simulink model "threeareaIPSnonlinear"  (R2018b)
settings: Solver=VariableStepAuto  StartTime=0.0  StopTime=100  RelTol=1e-3
values from neighbouring files (symbols this model uses):
  optim_param = Best_pos    [main.m]
  w1 = 0.001    [main.m]
  w2 = 0.001    [main.m]
undefined symbols (not defined in the file or in its folder): w3
settings Model: Creator=Orka  LastModifiedBy=Orka
settings SolverCC: ZeroCrossAlgorithm=Adaptive
settings DebuggingCC: MaskedZcDiagnostic=none  IgnoredZcDiagnostic=none

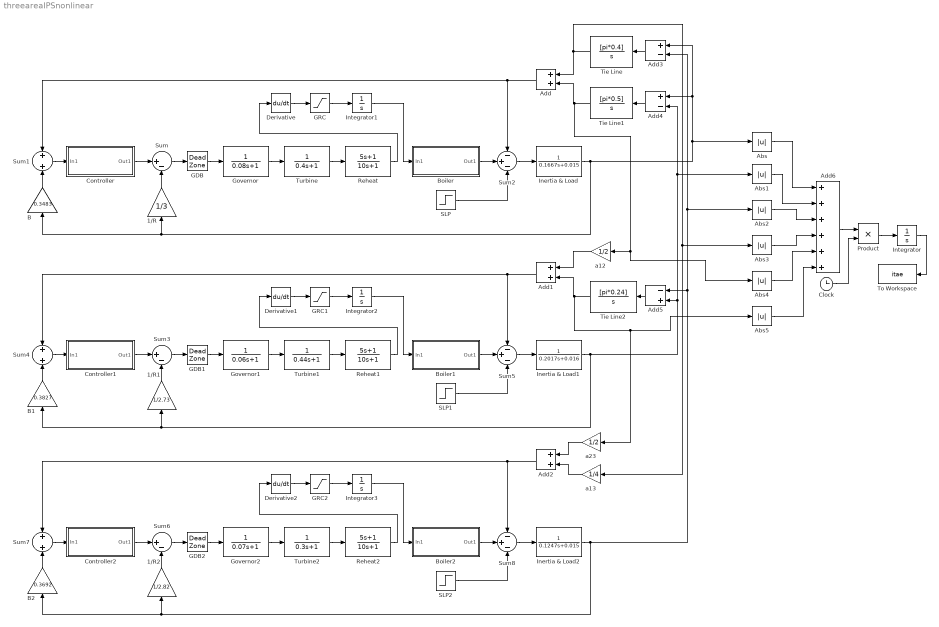
== system threeareaIPSnonlinear ==
  1/R : Gain  Gain=1/3
  1/R1 : Gain  Gain=1/2.73
  1/R2 : Gain  Gain=1/2.82
  Abs{,1..5} (6 alike) : Abs
  Add : Sum
  Add1 : Sum
  Add2 : Sum
  Add3 : Sum  Inputs=+-
  Add4 : Sum  Inputs=+-
  Add5 : Sum  Inputs=-+
  Add6 : Sum  Inputs=++++++
  B : Gain  Gain=0.3483
  B1 : Gain  Gain=0.3827
  B2 : Gain  Gain=0.3692
  Boiler : Subsystem
  Boiler1 : Subsystem
  Boiler2 : Subsystem
  Clock : Clock
  Controller : Subsystem
  Controller1 : Subsystem
  Controller2 : Subsystem
  Derivative : Derivative
  Derivative1 : Derivative
  Derivative2 : Derivative
  GDB : DeadZone  LowerValue=-0.036  UpperValue=0.036  SaturateOnIntegerOverflow=on
  GDB1 : DeadZone  LowerValue=-0.036  UpperValue=0.036  SaturateOnIntegerOverflow=on
  GDB2 : DeadZone  LowerValue=-0.036  UpperValue=0.036  SaturateOnIntegerOverflow=on
  GRC : Saturate  UpperLimit=0.0005  LowerLimit=-0.0005
  GRC1 : Saturate  UpperLimit=0.0005  LowerLimit=-0.0005
  GRC2 : Saturate  UpperLimit=0.0005  LowerLimit=-0.0005
  Governor : TransferFcn  Denominator=[0.08 1]
  Governor1 : TransferFcn  Denominator=[0.06 1]
  Governor2 : TransferFcn  Denominator=[0.07 1]
  Inertia & Load : TransferFcn  Denominator=[0.1667 0.015]
  Inertia & Load1 : TransferFcn  Denominator=[0.2017 0.016]
  Inertia & Load2 : TransferFcn  Denominator=[0.1247 0.015]
  Integrator{,1..3} (4 alike) : Integrator
  Product : Product
  Reheat : TransferFcn  Numerator=[5 1]  Denominator=[10 1]
  Reheat1 : TransferFcn  Numerator=[5 1]  Denominator=[10 1]
  Reheat2 : TransferFcn  Numerator=[5 1]  Denominator=[10 1]
  SLP : Step  After=w1  SampleTime=0
  SLP1 : Step  After=w2  SampleTime=0
  SLP2 : Step  After=w3  SampleTime=0
  Sum : Sum  Inputs=|+-
  Sum1 : Sum
  Sum2 : Sum  Inputs=-+-
  Sum3 : Sum  Inputs=|+-
  Sum4 : Sum
  Sum5 : Sum  Inputs=-+-
  Sum6 : Sum  Inputs=|+-
  Sum7 : Sum
  Sum8 : Sum  Inputs=-+-
  Tie Line : TransferFcn  Numerator=[pi*0.4]  Denominator=[1 0]
  Tie Line1 : TransferFcn  Numerator=[pi*0.5]  Denominator=[1 0]
  Tie Line2 : TransferFcn  Numerator=[pi*0.24]  Denominator=[1 0]
  To Workspace : ToWorkspace  VariableName=itae  SampleTime=-1
  Turbine : TransferFcn  Denominator=[0.4 1]
  Turbine1 : TransferFcn  Denominator=[0.44 1]
  Turbine2 : TransferFcn  Denominator=[0.3 1]
  a12 : Gain  Gain=1/2
  a13 : Gain  Gain=1/4
  a23 : Gain  Gain=1/2
  wires:
  GDB/1 -> Governor/1
  Governor/1 -> Turbine/1
  Turbine/1 -> Reheat/1
  Reheat/1 -> Derivative/1
  Derivative/1 -> GRC/1
  GRC/1 -> Integrator1/1
  Integrator1/1 -> Boiler/1(In1)
  Sum/1 -> GDB/1
  Controller/1(Out1) -> Sum/1
  1/R/1 -> Sum/2
  B/1 -> Sum1/2
  Boiler/1(Out1) -> Sum2/2
  SLP/1 -> Sum2/3
  Sum2/1 -> Inertia & Load/1
  Add/1 -> Sum2/1, Sum1/1
  Sum3/1 -> GDB1/1
  GDB1/1 -> Governor1/1
  Turbine1/1 -> Reheat1/1
  Derivative1/1 -> GRC1/1
  Boiler1/1(Out1) -> Sum5/2
  GRC1/1 -> Integrator2/1
  Sum5/1 -> Inertia & Load1/1
  SLP1/1 -> Sum5/3
  Add1/1 -> Sum5/1, Sum4/1
  Controller1/1(Out1) -> Sum3/1
  Governor1/1 -> Turbine1/1
  Reheat1/1 -> Derivative1/1
  Integrator2/1 -> Boiler1/1(In1)
  B1/1 -> Sum4/2
  1/R1/1 -> Sum3/2
  Sum6/1 -> GDB2/1
  GDB2/1 -> Governor2/1
  Turbine2/1 -> Reheat2/1
  Derivative2/1 -> GRC2/1
  Boiler2/1(Out1) -> Sum8/2
  GRC2/1 -> Integrator3/1
  Sum8/1 -> Inertia & Load2/1
  SLP2/1 -> Sum8/3
  Add2/1 -> Sum8/1, Sum7/1
  Controller2/1(Out1) -> Sum6/1
  Governor2/1 -> Turbine2/1
  Reheat2/1 -> Derivative2/1
  Integrator3/1 -> Boiler2/1(In1)
  B2/1 -> Sum7/2
  1/R2/1 -> Sum6/2
  a23/1 -> Add2/1
  a13/1 -> Add2/2
  Tie Line/1 -> Abs3/1, a13/1, Add/1
  Tie Line1/1 -> Abs4/1, a12/1, Add/2
  a12/1 -> Add1/1
  Tie Line2/1 -> Abs5/1, a23/1, Add1/2
  Add3/1 -> Tie Line/1
  Add4/1 -> Tie Line1/1
  Add5/1 -> Tie Line2/1
  Inertia & Load2/1 -> 1/R2/1, B2/1, Add5/1, Abs2/1, Add3/2
  Inertia & Load1/1 -> Abs1/1, Add4/2, Add5/2, 1/R1/1, B1/1
  Inertia & Load/1 -> 1/R/1, B/1, Abs/1, Add4/1, Add3/1
  Sum1/1 -> Controller/1(In1)
  Sum4/1 -> Controller1/1(In1)
  Sum7/1 -> Controller2/1(In1)
  Abs/1 -> Add6/1
  Abs1/1 -> Add6/2
  Abs2/1 -> Add6/3
  Abs3/1 -> Add6/4
  Abs4/1 -> Add6/5
  Abs5/1 -> Add6/6
  Add6/1 -> Product/1
  Clock/1 -> Product/2
  Product/1 -> Integrator/1
  Integrator/1 -> To Workspace/1

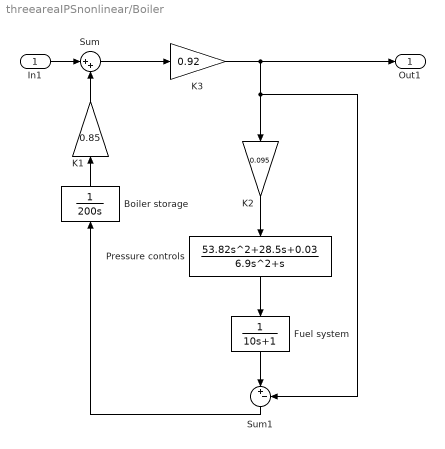
== system threeareaIPSnonlinear/Boiler ==
  In1 : Inport
  "  Boiler storage" : TransferFcn  Denominator=[200 0]
  Fuel system : TransferFcn  Denominator=[10 1]
  K1 : Gain  Gain=0.85
  K2 : Gain  Gain=0.095
  "K3 " : Gain  Gain=0.92
  "Pressure controls " : TransferFcn  Numerator=[53.82 28.5 0.03]  Denominator=[6.9 1 0]
  Sum : Sum  Inputs=|++
  Sum1 : Sum  Inputs=|+-
  Out1 : Outport
  wires:
  "  Boiler storage"/1 -> K1/1
  "Pressure controls "/1 -> Fuel system/1
  Sum1/1 -> "  Boiler storage"/1
  K1/1 -> Sum/2
  Sum/1 -> "K3 "/1
  Fuel system/1 -> Sum1/1
  K2/1 -> "Pressure controls "/1
  "K3 "/1 -> Out1/1, Sum1/2, K2/1
  In1/1 -> Sum/1

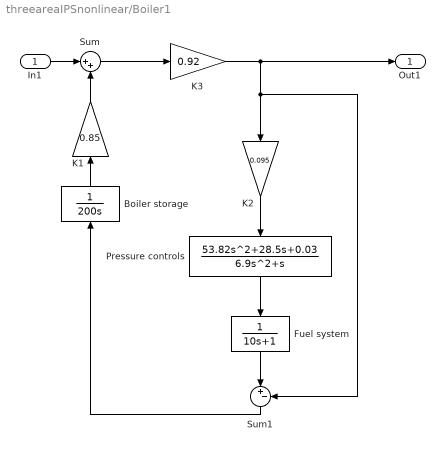
== system threeareaIPSnonlinear/Boiler1 ==
  In1 : Inport
  "  Boiler storage" : TransferFcn  Denominator=[200 0]
  Fuel system : TransferFcn  Denominator=[10 1]
  K1 : Gain  Gain=0.85
  K2 : Gain  Gain=0.095
  "K3 " : Gain  Gain=0.92
  "Pressure controls " : TransferFcn  Numerator=[53.82 28.5 0.03]  Denominator=[6.9 1 0]
  Sum : Sum  Inputs=|++
  Sum1 : Sum  Inputs=|+-
  Out1 : Outport
  wires:
  "  Boiler storage"/1 -> K1/1
  "Pressure controls "/1 -> Fuel system/1
  Sum1/1 -> "  Boiler storage"/1
  K1/1 -> Sum/2
  Sum/1 -> "K3 "/1
  Fuel system/1 -> Sum1/1
  K2/1 -> "Pressure controls "/1
  "K3 "/1 -> Out1/1, Sum1/2, K2/1
  In1/1 -> Sum/1

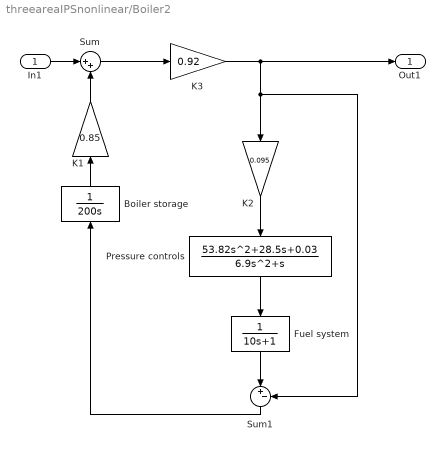
== system threeareaIPSnonlinear/Boiler2 ==
  In1 : Inport
  "  Boiler storage" : TransferFcn  Denominator=[200 0]
  Fuel system : TransferFcn  Denominator=[10 1]
  K1 : Gain  Gain=0.85
  K2 : Gain  Gain=0.095
  "K3 " : Gain  Gain=0.92
  "Pressure controls " : TransferFcn  Numerator=[53.82 28.5 0.03]  Denominator=[6.9 1 0]
  Sum : Sum  Inputs=|++
  Sum1 : Sum  Inputs=|+-
  Out1 : Outport
  wires:
  "  Boiler storage"/1 -> K1/1
  "Pressure controls "/1 -> Fuel system/1
  Sum1/1 -> "  Boiler storage"/1
  K1/1 -> Sum/2
  Sum/1 -> "K3 "/1
  Fuel system/1 -> Sum1/1
  K2/1 -> "Pressure controls "/1
  "K3 "/1 -> Out1/1, Sum1/2, K2/1
  In1/1 -> Sum/1

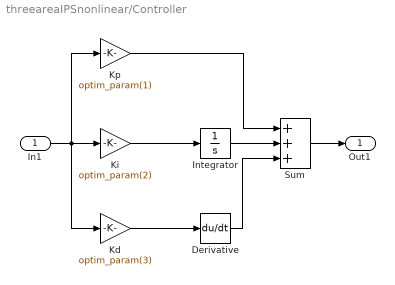
== system threeareaIPSnonlinear/Controller ==
  In1 : Inport
  Derivative : Derivative
  Integrator : Integrator
  Kd : Gain  Gain=optim_param(3)
  Ki : Gain  Gain=optim_param(2)
  Kp : Gain  Gain=optim_param(1)
  Sum : Sum  Inputs=+++
  Out1 : Outport
  wires:
  Sum/1 -> Out1/1
  Integrator/1 -> Sum/2
  Ki/1 -> Integrator/1
  Kd/1 -> Derivative/1
  Derivative/1 -> Sum/3
  In1/1 -> Kd/1, Kp/1, Ki/1
  Kp/1 -> Sum/1

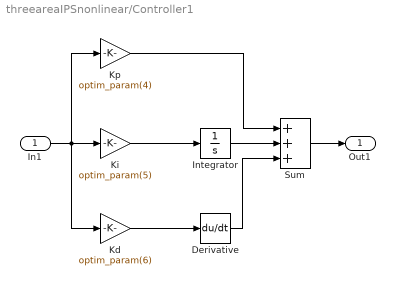
== system threeareaIPSnonlinear/Controller1 ==
  In1 : Inport
  Derivative : Derivative
  Integrator : Integrator
  Kd : Gain  Gain=optim_param(6)
  Ki : Gain  Gain=optim_param(5)
  Kp : Gain  Gain=optim_param(4)
  Sum : Sum  Inputs=+++
  Out1 : Outport
  wires:
  Sum/1 -> Out1/1
  Integrator/1 -> Sum/2
  Ki/1 -> Integrator/1
  Kd/1 -> Derivative/1
  Derivative/1 -> Sum/3
  In1/1 -> Kd/1, Kp/1, Ki/1
  Kp/1 -> Sum/1

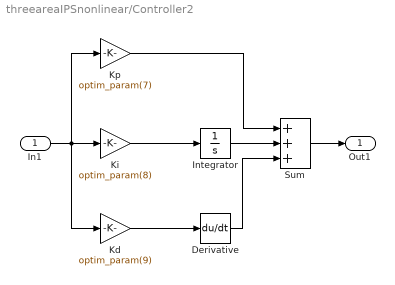
== system threeareaIPSnonlinear/Controller2 ==
  In1 : Inport
  Derivative : Derivative
  Integrator : Integrator
  Kd : Gain  Gain=optim_param(9)
  Ki : Gain  Gain=optim_param(8)
  Kp : Gain  Gain=optim_param(7)
  Sum : Sum  Inputs=+++
  Out1 : Outport
  wires:
  Sum/1 -> Out1/1
  Integrator/1 -> Sum/2
  Ki/1 -> Integrator/1
  Kd/1 -> Derivative/1
  Derivative/1 -> Sum/3
  In1/1 -> Kd/1, Kp/1, Ki/1
  Kp/1 -> Sum/1
